simulink model "cds_blockschaltbild_PT2"  (R2017b)
settings: Solver=ode45  StartTime=0.0  StopTime=10.0  MaxStep=1e-3  RelTol=1e-3  EnableMultiTasking=on
undefined symbols (not defined in the file or in its folder): A, B, C, D, G_tf, T, Ta, V, xi
libraries: cstblocks x2, simulink x1
settings Model: Creator=tk  LastModifiedBy=rbr
settings DataIOCC: LimitDataPoints=on  SaveFormat=Array  SignalLoggingSaveFormat=ModelDataLogs
settings OptimizationCC: ExpressionDepthLimit=2147483647  InitFltsAndDblsToZero=on  LifeSpan=inf
settings DebuggingCC: SaveWithParameterizedLinksMsg=none  UnderspecifiedInitializationDetection=Classic  MergeDetectMultiDrivingBlocksExec=none  SolverPrmCheckMsg=warning  StateNameClashWarn=warning  SFUnexpectedBacktrackingDiag=warning  SFNoUnconditionalDefaultTransitionDiag=warning  SFExecutionAtInitializationDiag=none
settings HardwareCC: ProdBitPerPointer=32  ProdBitPerSizeT=32  ProdBitPerPtrDiffT=32  ProdLargestAtomicFloat=None  ProdIntDivRoundTo=Undefined  ProdEndianess=Unspecified  ProdWordSize=32  ProdHWDeviceType=32-bit Generic
settings ModelReferenceCC: PropagateSignalLabelsOutOfModel=off
settings CodeAppCC: StateflowObjectComments=on
settings GRTTargetCC: TargetLangStandard=C89/C90 (ANSI)  GeneratePreprocessorConditionals=Disable all  CombineOutputUpdateFcns=off  GRTInterface=on
settings ConfigComp: CovMetricSettings=dw  CovHtmlReporting=on  CovSaveCumulativeToWorkspaceVar=on  CovSaveSingleToWorkspaceVar=on  CovExternalEMLEnable=off

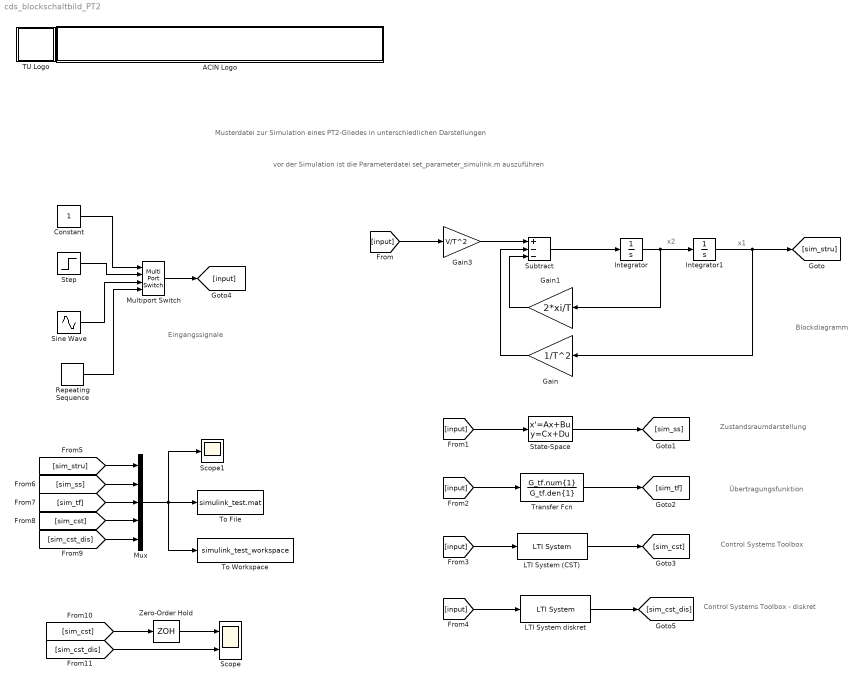
== system cds_blockschaltbild_PT2 ==
  note: x2
  note: x1
  note: Musterdatei zur Simulation eines PT2-Gliedes in unterschiedlichen Darstellungen
  note: Blockdiagramm
  note: Zustandsraumdarstellung
  note: Übertragungsfunktion
  note: Control Systems Toolbox
  note: Control Systems Toolbox - diskret
  note: vor der Simulation ist die Parameterdatei set_parameter_simulink.m auszuführen
  note: Eingangssignale
  ACIN Logo : Subsystem
      mask init:
      | s = get_param(gcb,'UserData');
      mask Display:
      | image(s.logo,[0 0 439 45]);
      | %axis image
  Constant : Constant
  Gain : Gain  Gain=1/T^2
  Gain1 : Gain  Gain=2*xi/T
  Gain3 : Gain  Gain=V/T^2
  Integrator : Integrator
  Integrator1 : Integrator
  LTI System (CST) : cstblocks/LTI System  sys=sys  IC=[]
  LTI System diskret : cstblocks/LTI System  sys=G_z  IC=[]
  Multiport Switch : MultiPortSwitch
  Mux : Mux  Inputs=5
  Repeating Sequence : simulink/Sources/Repeating Sequence  rep_seq_t=[0 2]  rep_seq_y=[0 2]
  Scope : Scope  NumInputPorts=2
  Scope1 : Scope
  Sine Wave : Sin  SampleTime=0
  State-Space : StateSpace  A=A  B=B  C=C  D=D  InitialCondition=0
  Step : Step  SampleTime=0
  Subtract : Sum  Inputs=+--
  TU Logo : Subsystem
      mask init:
      | s = get_param(gcb,'UserData');
      mask Display: image(s.logo,[0 0 45 45]);
  To File : ToFile  Filename=simulink_test.mat
  To Workspace : ToWorkspace  VariableName=simulink_test_workspace  SaveFormat=Structure With Time  SampleTime=-1
  Transfer Fcn : TransferFcn  Numerator=G_tf.num{1}  Denominator=G_tf.den{1}
  Zero-Order Hold : ZeroOrderHold  SampleTime=Ta
  wires:
  Subtract/1 -> Integrator/1
  Integrator/1 -> Integrator1/1, Gain1/1
  Gain1/1 -> Subtract/3
  Gain/1 -> Subtract/2
  Integrator1/1 -> Gain/1, [sim_stru]
  Gain3/1 -> Subtract/1
  Constant/1 -> Multiport Switch/1
  Step/1 -> Multiport Switch/2
  Sine Wave/1 -> Multiport Switch/3
  Repeating Sequence/1 -> Multiport Switch/4
  Multiport Switch/1 -> [input]
  [input] -> Gain3/1
  [input] -> State-Space/1
  [input] -> Transfer Fcn/1
  [input] -> LTI System (CST)/1
  State-Space/1 -> [sim_ss]
  Transfer Fcn/1 -> [sim_tf]
  LTI System (CST)/1 -> [sim_cst]
  [input] -> LTI System diskret/1
  LTI System diskret/1 -> [sim_cst_dis]
  [sim_stru] -> Mux/1
  [sim_ss] -> Mux/2
  [sim_tf] -> Mux/3
  [sim_cst] -> Mux/4
  [sim_cst_dis] -> Mux/5
  Mux/1 -> To File/1, To Workspace/1, Scope1/1
  [sim_cst] -> Zero-Order Hold/1
  [sim_cst_dis] -> Scope/2
  Zero-Order Hold/1 -> Scope/1

== system cds_blockschaltbild_PT2/ACIN Logo ==

== system cds_blockschaltbild_PT2/TU Logo ==
